simulink model "Complex_Throttle_Regime"  (R2024b)
settings: Solver=VariableStepAuto  StartTime=0.0  StopTime=525  RelTol=1e-3
libraries: Solver_SF x1
settings Model: Creator=Pain  LastModifiedBy=Pain

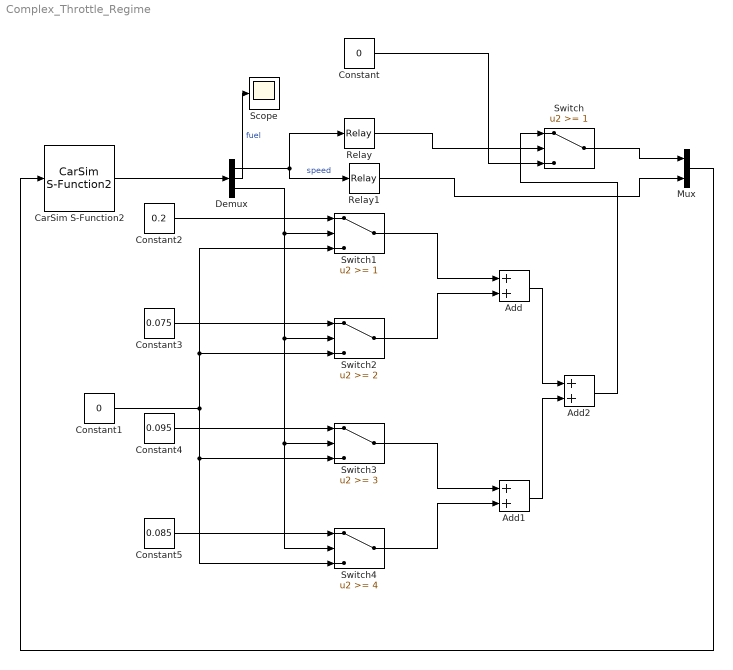
== system Complex_Throttle_Regime ==
  Add : Sum
  Add1 : Sum
  Add2 : Sum
  CarSim S-Function2 : Solver_SF/CarSim S-Function2  Priority=1  VehicleCode=i_i  SIMFILE=simfile.sim
      settings: AttributesFormatString=Vehicle Code: %<VehicleCode>  SourceProductName=CarSim S-Function
  Constant : Constant  Value=0
  Constant1 : Constant  Value=0
  Constant2 : Constant  Value=0.2
  Constant3 : Constant  Value=0.075
  Constant4 : Constant  Value=0.095
  Constant5 : Constant  Value=0.085
  Demux : Demux  Outputs=3
  Mux : Mux  Inputs=2
  Relay : Relay  OnSwitchValue=35  OffSwitchValue=15  OnOutputValue=0  OffOutputValue=1
  Relay1 : Relay  OnSwitchValue=35  OffSwitchValue=15
  Scope : Scope
  Switch : Switch  Threshold=1  SaturateOnIntegerOverflow=off  InputSameDT=off
  Switch1 : Switch  Threshold=1  SaturateOnIntegerOverflow=off  InputSameDT=off
  Switch2 : Switch  Threshold=2  SaturateOnIntegerOverflow=off  InputSameDT=off
  Switch3 : Switch  Threshold=3  SaturateOnIntegerOverflow=off  InputSameDT=off
  Switch4 : Switch  Threshold=4  SaturateOnIntegerOverflow=off  InputSameDT=off
  wires:
  CarSim S-Function2/1 -> Demux/1
  Relay/1 -> Switch/2
  Demux/1 -> Relay/1, Relay1/1  "speed"
  Demux/3 -> Switch4/2, Switch3/2, Switch2/2, Switch1/2
  Constant1/1 -> Switch1/3, Switch2/3, Switch3/3, Switch4/3
  Constant2/1 -> Switch1/1
  Constant3/1 -> Switch2/1
  Switch1/1 -> Add/1
  Switch2/1 -> Add/2
  Switch3/1 -> Add1/1
  Switch4/1 -> Add1/2
  Add/1 -> Add2/1
  Add1/1 -> Add2/2
  Demux/2 -> Scope/1  "fuel"
  Switch/1 -> Mux/1
  Relay1/1 -> Mux/2
  Mux/1 -> CarSim S-Function2/1
  Constant4/1 -> Switch3/1
  Constant5/1 -> Switch4/1
  Constant/1 -> Switch/3
  Add2/1 -> Switch/1
